simulink library "TOS_LIB"  (R2019b)
settings: Solver=VariableStepAuto  StartTime=0.0  StopTime=10.0  RelTol=1e-3
undefined symbols (not defined in the file): AEBSFunctionLib, Data, Prob_Filt
libraries: simulink x27
settings Model: Creator=GW00157303  LastModifiedBy=GW00115634
settings DataIOCC: ReturnWorkspaceOutputs=off
settings DebuggingCC: ArithmeticOperatorsInVariantConditions=warning
settings SFSimCC: SimUseLocalCustomCode=off  CustomCodeUndefinedFunction=UseInterfaceOnly
settings RTWCC: RTWUseLocalCustomCode=off
settings CodeAppCC: StateflowObjectComments=on

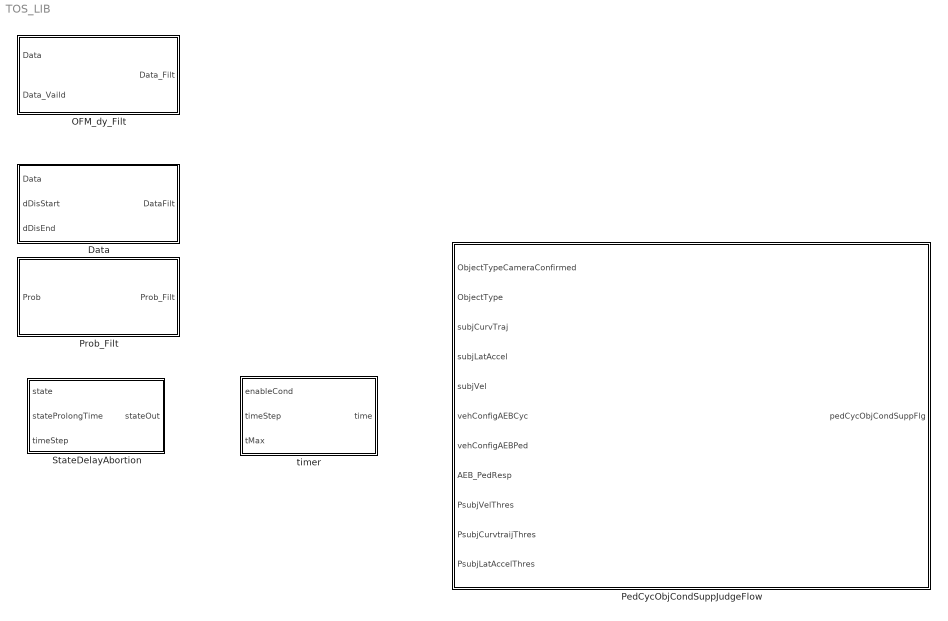
== system TOS_LIB ==
  Data : Subsystem  AncestorBlock=AEBSFunctionLib/Data
  OFM_dy_Filt : Subsystem  AncestorBlock=TOS_LIB/Prob_Filt
  PedCycObjCondSuppJudgeFlow : Subsystem  TreatAsAtomicUnit=on
  Prob_Filt : Subsystem  AncestorBlock=AEBSFunctionLib/Prob_Filt
  StateDelayAbortion : Subsystem  TreatAsAtomicUnit=on
  timer : Subsystem  TreatAsAtomicUnit=on

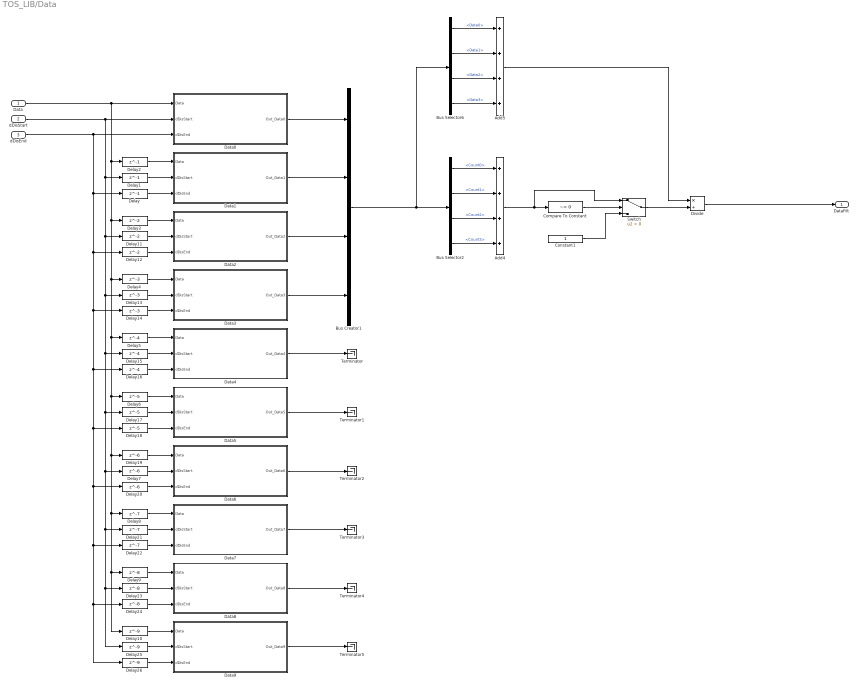
== system TOS_LIB/Data ==
  Data : Inport
  dDisStart : Inport  Port=2
  dDisEnd : Inport  Port=3
  Add4 : Sum  Inputs=++++
  Add5 : Sum  Inputs=++++
  Bus Creator1 : BusCreator  Inputs=4
  Bus Selector2 : BusSelector  OutputSignals=Out_Data0.Count0,Out_Data1.Count1,Out_Data2.Count2,Out_Data3.Count3
  Bus Selector6 : BusSelector  OutputSignals=Out_Data0.Data0,Out_Data1.Data1,Out_Data2.Data2,Out_Data3.Data3
  Compare To Constant : simulink/Logic and Bit Operations/Compare To Constant  relop=~=  const=0  OutDataTypeStr=boolean
  Constant1 : Constant  OutDataTypeStr=single
  Data0 : Subsystem
  Data1 : Subsystem
  Data2 : Subsystem
  Data3 : Subsystem
  Data4 : Subsystem
  Data5 : Subsystem
  Data6 : Subsystem
  Data7 : Subsystem
  Data8 : Subsystem
  Data9 : Subsystem
  Delay : Delay  DelayLength=1  InitialCondition=0
  Delay1 : Delay  DelayLength=1  InitialCondition=0
  Delay10 : Delay  DelayLength=9  InitialCondition=0
  Delay11 : Delay  InitialCondition=0
  Delay12 : Delay  InitialCondition=0
  Delay13 : Delay  DelayLength=3  InitialCondition=0
  Delay14 : Delay  DelayLength=3  InitialCondition=0
  Delay15 : Delay  DelayLength=4  InitialCondition=0
  Delay16 : Delay  DelayLength=4  InitialCondition=0
  Delay17 : Delay  DelayLength=5  InitialCondition=0
  Delay18 : Delay  DelayLength=5  InitialCondition=0
  Delay19 : Delay  DelayLength=6  InitialCondition=0
  Delay2 : Delay  DelayLength=1  InitialCondition=0
  Delay20 : Delay  DelayLength=6  InitialCondition=0
  Delay21 : Delay  DelayLength=7  InitialCondition=0
  Delay22 : Delay  DelayLength=7  InitialCondition=0
  Delay23 : Delay  DelayLength=8  InitialCondition=0
  Delay24 : Delay  DelayLength=8  InitialCondition=0
  Delay25 : Delay  DelayLength=9  InitialCondition=0
  Delay26 : Delay  DelayLength=9  InitialCondition=0
  Delay3 : Delay  InitialCondition=0
  Delay4 : Delay  DelayLength=3  InitialCondition=0
  Delay5 : Delay  DelayLength=4  InitialCondition=0
  Delay6 : Delay  DelayLength=5  InitialCondition=0
  Delay7 : Delay  DelayLength=6  InitialCondition=0
  Delay8 : Delay  DelayLength=7  InitialCondition=0
  Delay9 : Delay  DelayLength=8  InitialCondition=0
  Divide : Product  Inputs=*/
  Switch : Switch  Criteria=u2 > Threshold
  Terminator{,1..5} (6 alike) : Terminator
  DataFilt : Outport
  wires:
  Delay21/1 -> Data7/2(dDisStart)
  Delay18/1 -> Data5/3(dDisEnd)
  Delay9/1 -> Data8/1(Data)
  Delay22/1 -> Data7/3(dDisEnd)
  Delay23/1 -> Data8/2(dDisStart)
  Delay26/1 -> Data9/3(dDisEnd)
  Delay4/1 -> Data3/1(Data)
  Add5/1 -> Divide/1
  Delay12/1 -> Data2/3(dDisEnd)
  Delay8/1 -> Data7/1(Data)
  Data9/1(Out_Data9) -> Terminator5/1
  Data1/1(Out_Data1) -> Bus Creator1/2
  Delay7/1 -> Data6/2(dDisStart)
  dDisEnd/1 -> Data0/3(dDisEnd), Delay16/1, Delay20/1, Delay22/1, Delay26/1, Delay24/1, Delay18/1, Delay14/1, Delay12/1, Delay/1
  Delay19/1 -> Data6/1(Data)
  Delay13/1 -> Data3/2(dDisStart)
  Switch/1 -> Divide/2
  Delay14/1 -> Data3/3(dDisEnd)
  Data7/1(Out_Data7) -> Terminator3/1
  Add4/1 -> Compare To Constant/1, Switch/1
  Delay25/1 -> Data9/2(dDisStart)
  Divide/1 -> DataFilt/1
  Delay10/1 -> Data9/1(Data)
  Delay6/1 -> Data5/1(Data)
  Data4/1(Out_Data4) -> Terminator/1
  Compare To Constant/1 -> Switch/2
  Delay17/1 -> Data5/2(dDisStart)
  Delay2/1 -> Data1/1(Data)
  Delay5/1 -> Data4/1(Data)
  Delay3/1 -> Data2/1(Data)
  Delay/1 -> Data1/3(dDisEnd)
  Data3/1(Out_Data3) -> Bus Creator1/4
  Delay20/1 -> Data6/3(dDisEnd)
  Data8/1(Out_Data8) -> Terminator4/1
  Delay24/1 -> Data8/3(dDisEnd)
  dDisStart/1 -> Data0/2(dDisStart), Delay1/1, Delay25/1, Delay23/1, Delay21/1, Delay7/1, Delay17/1, Delay15/1, Delay13/1, Delay11/1
  Bus Creator1/1 -> Bus Selector2/1, Bus Selector6/1
  Data6/1(Out_Data6) -> Terminator2/1
  Delay1/1 -> Data1/2(dDisStart)
  Data5/1(Out_Data5) -> Terminator1/1
  Delay16/1 -> Data4/3(dDisEnd)
  Data2/1(Out_Data2) -> Bus Creator1/3
  Constant1/1 -> Switch/3
  Delay15/1 -> Data4/2(dDisStart)
  Data0/1(Out_Data0) -> Bus Creator1/1
  Delay11/1 -> Data2/2(dDisStart)
  Data/1 -> Delay2/1, Delay3/1, Delay6/1, Delay19/1, Delay8/1, Delay9/1, Delay10/1, Delay5/1, Delay4/1, Data0/1(Data)
  Bus Selector6/1 -> Add5/1  "<Data0>"
  Bus Selector6/2 -> Add5/2  "<Data1>"
  Bus Selector6/3 -> Add5/3  "<Data2>"
  Bus Selector6/4 -> Add5/4  "<Data3>"
  Bus Selector2/1 -> Add4/1  "<Count0>"
  Bus Selector2/2 -> Add4/2  "<Count1>"
  Bus Selector2/3 -> Add4/3  "<Count2>"
  Bus Selector2/4 -> Add4/4  "<Count3>"

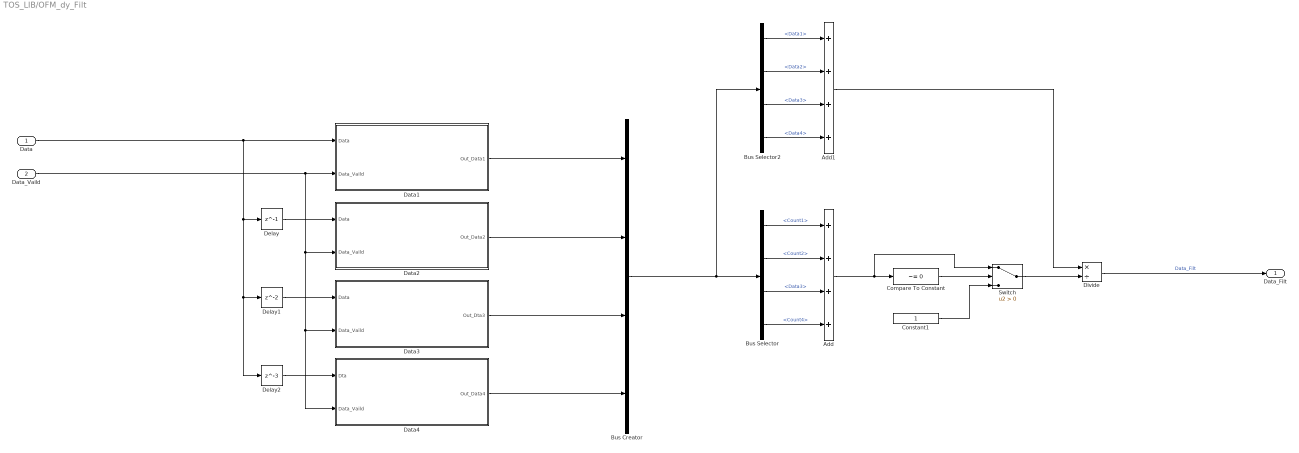
== system TOS_LIB/OFM_dy_Filt ==
  Data : Inport
  Data_Vaild : Inport  Port=2
  Add : Sum  Inputs=++++
  Add1 : Sum  Inputs=++++
  Bus Creator : BusCreator  Inputs=4
  Bus Selector : BusSelector  OutputSignals=Out_Data1.Count1,Out_Data2.Count2,Out_Data3.Data3,Out_Data4.Count4
  Bus Selector2 : BusSelector  OutputSignals=Out_Data1.Data1,Out_Data2.Data2,Out_Data3.Data3,Out_Data4.Data4
  Compare To Constant : simulink/Logic and Bit Operations/Compare To Constant  relop=~=  const=0  OutDataTypeStr=boolean
  Constant1 : Constant  OutDataTypeStr=single
  Data1 : Subsystem
  Data2 : Subsystem
  Data3 : Subsystem
  Data4 : Subsystem
  Delay : Delay  DelayLength=1  InitialCondition=0
  Delay1 : Delay  InitialCondition=0
  Delay2 : Delay  DelayLength=3  InitialCondition=0
  Divide : Product  Inputs=*/
  Switch : Switch  Criteria=u2 > Threshold
  Data_Filt : Outport
  wires:
  Bus Selector/4 -> Add/4  "<Count4>"
  Bus Selector/3 -> Add/3  "<Data3>"
  Bus Selector/2 -> Add/2  "<Count2>"
  Bus Selector/1 -> Add/1  "<Count1>"
  Bus Selector2/4 -> Add1/4  "<Data4>"
  Bus Selector2/3 -> Add1/3  "<Data3>"
  Bus Selector2/2 -> Add1/2  "<Data2>"
  Bus Selector2/1 -> Add1/1  "<Data1>"
  Divide/1 -> Data_Filt/1  "Data_Filt"
  Data3/1(Out_Dta3) -> Bus Creator/3
  Add1/1 -> Divide/1
  Data/1 -> Delay2/1, Delay1/1, Delay/1, Data1/1(Data)
  Delay2/1 -> Data4/1(Dta)
  Delay/1 -> Data2/1(Data)
  Data1/1(Out_Data1) -> Bus Creator/1
  Data2/1(Out_Data2) -> Bus Creator/2
  Bus Creator/1 -> Bus Selector2/1, Bus Selector/1
  Compare To Constant/1 -> Switch/2
  Constant1/1 -> Switch/3
  Add/1 -> Switch/1, Compare To Constant/1
  Delay1/1 -> Data3/1(Data)
  Data4/1(Out_Data4) -> Bus Creator/4
  Switch/1 -> Divide/2
  Data_Vaild/1 -> Data3/2(Data_Vaild), Data4/2(Data_Vaild), Data2/2(Data_Vaild), Data1/2(Data_Vaild)

== system TOS_LIB/PedCycObjCondSuppJudgeFlow ==
  ObjectTypeCameraConfirmed : Inport
  ObjectType : Inport  Port=2
  subjCurvTraj : Inport  Port=3
  subjLatAccel : Inport  Port=4
  subjVel : Inport  Port=5
  vehConfigAEBCyc : Inport  Port=6
  vehConfigAEBPed : Inport  Port=7
  AEB_PedResp : Inport  Port=8
  PsubjVelThres : Inport  Port=9
  PsubjCurvtraijThres : Inport  Port=10
  PsubjLatAccelThres : Inport  Port=11
  PedCycObjCondSuppJudgeFlow : Stateflow chart  TreatAsAtomicUnit=on
  pedCycObjCondSuppFlg : Outport
  wires:
  PsubjLatAccelThres/1 -> PedCycObjCondSuppJudgeFlow/11(PsubjLatAccelThres)
  PsubjCurvtraijThres/1 -> PedCycObjCondSuppJudgeFlow/10(PsubjCurvtraijThres)
  PedCycObjCondSuppJudgeFlow/1(pedCycObjCondSuppFlg) -> pedCycObjCondSuppFlg/1
  vehConfigAEBCyc/1 -> PedCycObjCondSuppJudgeFlow/6(vehConfigAEBCyc)
  subjLatAccel/1 -> PedCycObjCondSuppJudgeFlow/4(subjLatAccel)
  subjVel/1 -> PedCycObjCondSuppJudgeFlow/5(subjVel)
  ObjectType/1 -> PedCycObjCondSuppJudgeFlow/2(objType)
  AEB_PedResp/1 -> PedCycObjCondSuppJudgeFlow/8(AEB_PedResp)
  subjCurvTraj/1 -> PedCycObjCondSuppJudgeFlow/3(subjCurvTraj)
  vehConfigAEBPed/1 -> PedCycObjCondSuppJudgeFlow/7(vehConfigAEBPed)
  PsubjVelThres/1 -> PedCycObjCondSuppJudgeFlow/9(PsubjVelThres)
  ObjectTypeCameraConfirmed/1 -> PedCycObjCondSuppJudgeFlow/1(ObjectTypeCameraConfirmed)

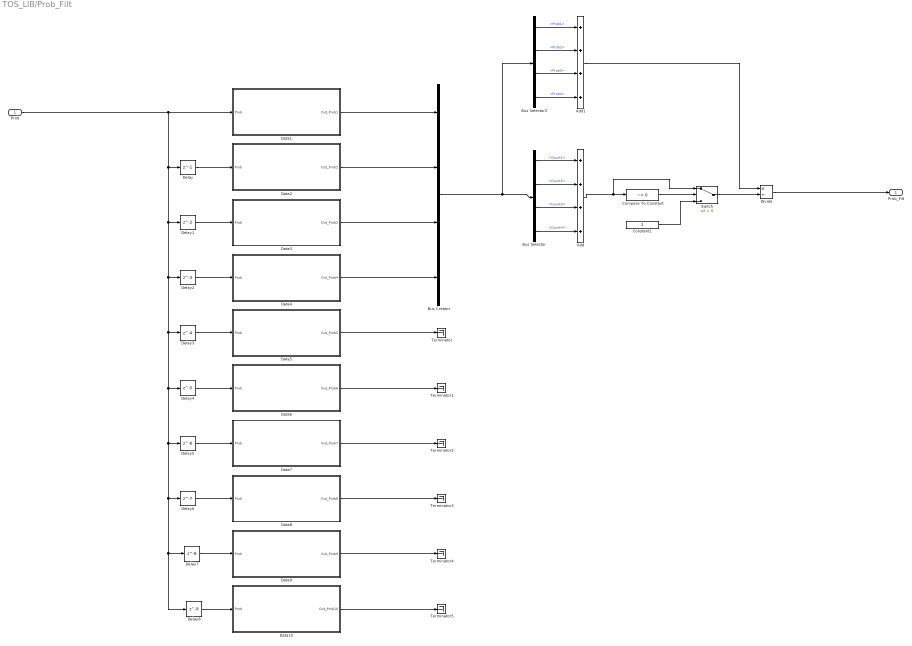
== system TOS_LIB/Prob_Filt ==
  Prob : Inport
  Add : Sum  Inputs=++++
  Add1 : Sum  Inputs=++++
  Bus Creator : BusCreator  Inputs=4
  Bus Selector : BusSelector  OutputSignals=Out_Prob1.Count1,Out_Prob2.Count2,Out_Prob3.Count3,Out_Prob4.Count4
  Bus Selector2 : BusSelector  OutputSignals=Out_Prob1.Prob1,Out_Prob2.Prob2,Out_Prob3.Prob3,Out_Prob4.Prob4
  Compare To Constant : simulink/Logic and Bit Operations/Compare To Constant  relop=~=  const=0  OutDataTypeStr=boolean
  Constant1 : Constant  OutDataTypeStr=single
  Data1 : Subsystem
  Data10 : Subsystem
  Data2 : Subsystem
  Data3 : Subsystem
  Data4 : Subsystem
  Data5 : Subsystem
  Data6 : Subsystem
  Data7 : Subsystem
  Data8 : Subsystem
  Data9 : Subsystem
  Delay : Delay  DelayLength=1  InitialCondition=0
  Delay1 : Delay  InitialCondition=0
  Delay2 : Delay  DelayLength=3  InitialCondition=0
  Delay3 : Delay  DelayLength=4  InitialCondition=0
  Delay4 : Delay  DelayLength=5  InitialCondition=0
  Delay5 : Delay  DelayLength=6  InitialCondition=0
  Delay6 : Delay  DelayLength=7  InitialCondition=0
  Delay7 : Delay  DelayLength=8  InitialCondition=0
  Delay8 : Delay  DelayLength=9  InitialCondition=0
  Divide : Product  Inputs=*/
  Switch : Switch  Criteria=u2 > Threshold
  Terminator{,1..5} (6 alike) : Terminator
  Prob_Filt : Outport
  wires:
  Switch/1 -> Divide/2
  Delay5/1 -> Data7/1(Prob)
  Delay3/1 -> Data5/1(Prob)
  Data4/1(Out_Prob4) -> Bus Creator/4
  Delay1/1 -> Data3/1(Prob)
  Delay8/1 -> Data10/1(Prob)
  Data8/1(Out_Prob8) -> Terminator3/1
  Add/1 -> Compare To Constant/1, Switch/1
  Constant1/1 -> Switch/3
  Delay6/1 -> Data8/1(Prob)
  Data10/1(Out_Prob10) -> Terminator5/1
  Compare To Constant/1 -> Switch/2
  Data5/1(Out_Prob5) -> Terminator/1
  Bus Creator/1 -> Bus Selector/1, Bus Selector2/1
  Data2/1(Out_Prob2) -> Bus Creator/2
  Data1/1(Out_Prob1) -> Bus Creator/1
  Data9/1(Out_Prob9) -> Terminator4/1
  Delay7/1 -> Data9/1(Prob)
  Delay4/1 -> Data6/1(Prob)
  Delay/1 -> Data2/1(Prob)
  Data6/1(Out_Prob6) -> Terminator1/1
  Data7/1(Out_Prob7) -> Terminator2/1
  Delay2/1 -> Data4/1(Prob)
  Prob/1 -> Delay1/1, Delay8/1, Delay7/1, Delay6/1, Delay5/1, Delay4/1, Delay3/1, Delay2/1, Delay/1, Data1/1(Prob)
  Add1/1 -> Divide/1
  Data3/1(Out_Prob3) -> Bus Creator/3
  Divide/1 -> Prob_Filt/1
  Bus Selector2/1 -> Add1/1  "<Prob1>"
  Bus Selector2/2 -> Add1/2  "<Prob2>"
  Bus Selector2/3 -> Add1/3  "<Prob3>"
  Bus Selector2/4 -> Add1/4  "<Prob4>"
  Bus Selector/1 -> Add/1  "<Count1>"
  Bus Selector/2 -> Add/2  "<Count2>"
  Bus Selector/3 -> Add/3  "<Count3>"
  Bus Selector/4 -> Add/4  "<Count4>"

== system TOS_LIB/StateDelayAbortion ==
  state : Inport
  stateProlongTime : Inport  Port=2
  timeStep : Inport  Port=3
  StateDelayAbortion : Stateflow chart  TreatAsAtomicUnit=on
  Terminator : Terminator
  Terminator1 : Terminator
  Unit Delay : UnitDelay  SampleTime=-1  HasFrameUpgradeWarning=on
  stateOut : Outport
  wires:
  StateDelayAbortion/2(stateOut) -> stateOut/1
  StateDelayAbortion/1(timeSinceLastState) -> Terminator/1  "timeSinceLastState"
  timeStep/1 -> StateDelayAbortion/4(Ts)
  stateProlongTime/1 -> StateDelayAbortion/3(stateProlongationTime)
  Unit Delay/1 -> StateDelayAbortion/2(stateK1)
  state/1 -> StateDelayAbortion/1(state), Unit Delay/1
  StateDelayAbortion/3(Flag) -> Terminator1/1  "Flag"

== system TOS_LIB/timer ==
  enableCond : Inport
  timeStep : Inport  Port=2
  tMax : Inport  Port=3
  If Action Subsystem2 : Subsystem  TreatAsAtomicUnit=on
  If Action Subsystem3 : Subsystem  TreatAsAtomicUnit=on
  If1 : If  IfExpression=u1
  Merge1 : Merge
  time : Outport
  wires:
  If1/1 -> If Action Subsystem2/Action
  If Action Subsystem2/1(time) -> Merge1/1
  If1/2 -> If Action Subsystem3/Action
  If Action Subsystem3/1(time) -> Merge1/2
  enableCond/1 -> If1/1
  timeStep/1 -> If Action Subsystem2/1(timeStep)
  Merge1/1 -> time/1  "time"
  tMax/1 -> If Action Subsystem2/2(tMax)

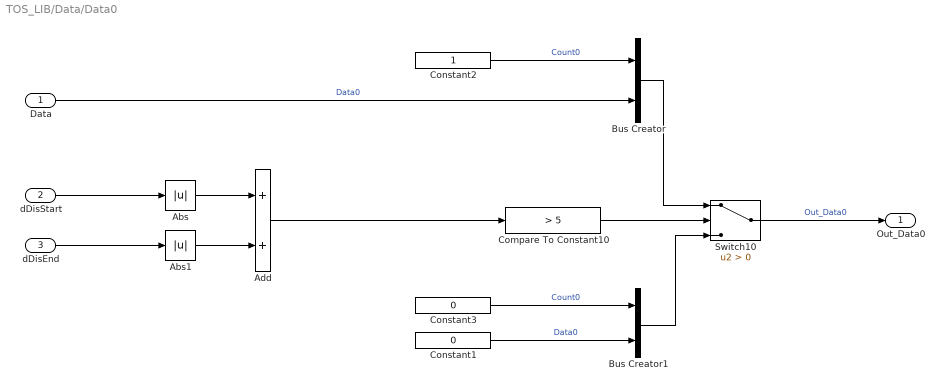
== system TOS_LIB/Data/Data0 ==
  Data : Inport
  dDisStart : Inport  Port=2
  dDisEnd : Inport  Port=3
  Abs : Abs
  Abs1 : Abs
  Add : Sum
  Bus Creator : BusCreator  Inputs=2
  Bus Creator1 : BusCreator  Inputs=2
  Compare To Constant10 : simulink/Logic and Bit Operations/Compare To Constant  relop=>  const=5  OutDataTypeStr=boolean
  Constant1 : Constant  Value=0  OutDataTypeStr=single
  Constant2 : Constant  OutDataTypeStr=uint8
  Constant3 : Constant  Value=0  OutDataTypeStr=uint8
  Switch10 : Switch  Criteria=u2 > Threshold
  Out_Data0 : Outport
  wires:
  Compare To Constant10/1 -> Switch10/2
  Constant3/1 -> Bus Creator1/1  "Count0"
  Constant1/1 -> Bus Creator1/2  "Data0"
  Switch10/1 -> Out_Data0/1  "Out_Data0"
  Constant2/1 -> Bus Creator/1  "Count0"
  Bus Creator1/1 -> Switch10/3
  Bus Creator/1 -> Switch10/1
  Add/1 -> Compare To Constant10/1
  dDisStart/1 -> Abs/1
  dDisEnd/1 -> Abs1/1
  Abs/1 -> Add/1
  Abs1/1 -> Add/2
  Data/1 -> Bus Creator/2  "Data0"

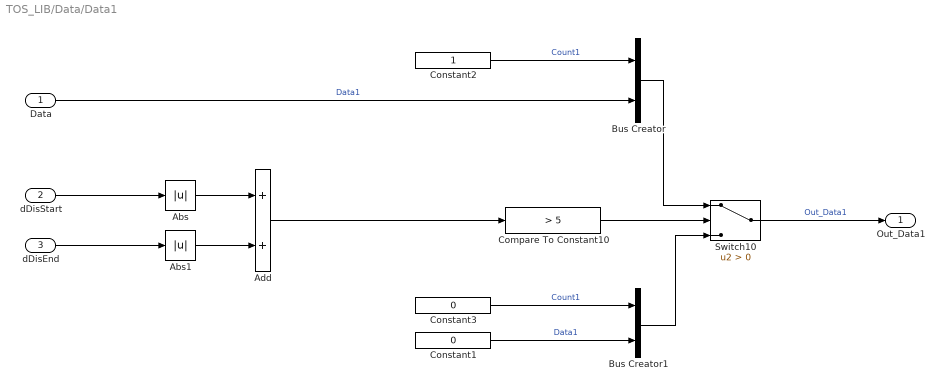
== system TOS_LIB/Data/Data1 ==
  Data : Inport
  dDisStart : Inport  Port=2
  dDisEnd : Inport  Port=3
  Abs : Abs
  Abs1 : Abs
  Add : Sum
  Bus Creator : BusCreator  Inputs=2
  Bus Creator1 : BusCreator  Inputs=2
  Compare To Constant10 : simulink/Logic and Bit Operations/Compare To Constant  relop=>  const=5  OutDataTypeStr=boolean
  Constant1 : Constant  Value=0  OutDataTypeStr=single
  Constant2 : Constant  OutDataTypeStr=uint8
  Constant3 : Constant  Value=0  OutDataTypeStr=uint8
  Switch10 : Switch  Criteria=u2 > Threshold
  Out_Data1 : Outport
  wires:
  Data/1 -> Bus Creator/2  "Data1"
  Abs1/1 -> Add/2
  Abs/1 -> Add/1
  dDisEnd/1 -> Abs1/1
  dDisStart/1 -> Abs/1
  Add/1 -> Compare To Constant10/1
  Bus Creator/1 -> Switch10/1
  Bus Creator1/1 -> Switch10/3
  Constant2/1 -> Bus Creator/1  "Count1"
  Switch10/1 -> Out_Data1/1  "Out_Data1"
  Constant1/1 -> Bus Creator1/2  "Data1"
  Constant3/1 -> Bus Creator1/1  "Count1"
  Compare To Constant10/1 -> Switch10/2

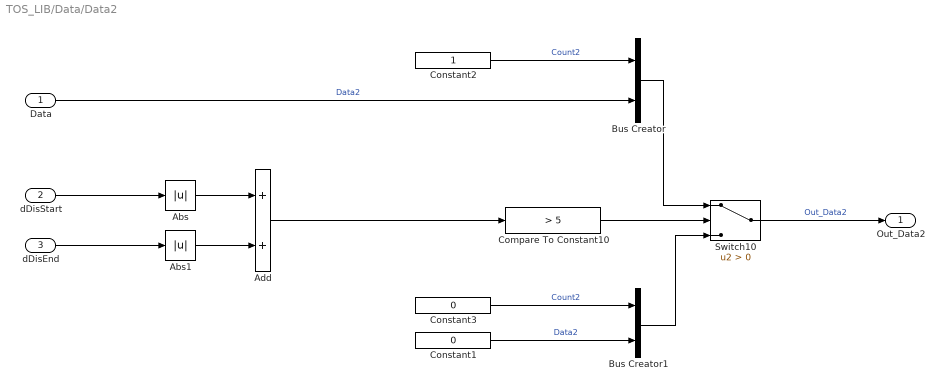
== system TOS_LIB/Data/Data2 ==
  Data : Inport
  dDisStart : Inport  Port=2
  dDisEnd : Inport  Port=3
  Abs : Abs
  Abs1 : Abs
  Add : Sum
  Bus Creator : BusCreator  Inputs=2
  Bus Creator1 : BusCreator  Inputs=2
  Compare To Constant10 : simulink/Logic and Bit Operations/Compare To Constant  relop=>  const=5  OutDataTypeStr=boolean
  Constant1 : Constant  Value=0  OutDataTypeStr=single
  Constant2 : Constant  OutDataTypeStr=uint8
  Constant3 : Constant  Value=0  OutDataTypeStr=uint8
  Switch10 : Switch  Criteria=u2 > Threshold
  Out_Data2 : Outport
  wires:
  Compare To Constant10/1 -> Switch10/2
  Constant3/1 -> Bus Creator1/1  "Count2"
  Constant1/1 -> Bus Creator1/2  "Data2"
  Switch10/1 -> Out_Data2/1  "Out_Data2"
  Constant2/1 -> Bus Creator/1  "Count2"
  Bus Creator1/1 -> Switch10/3
  Bus Creator/1 -> Switch10/1
  Add/1 -> Compare To Constant10/1
  dDisStart/1 -> Abs/1
  dDisEnd/1 -> Abs1/1
  Abs/1 -> Add/1
  Abs1/1 -> Add/2
  Data/1 -> Bus Creator/2  "Data2"

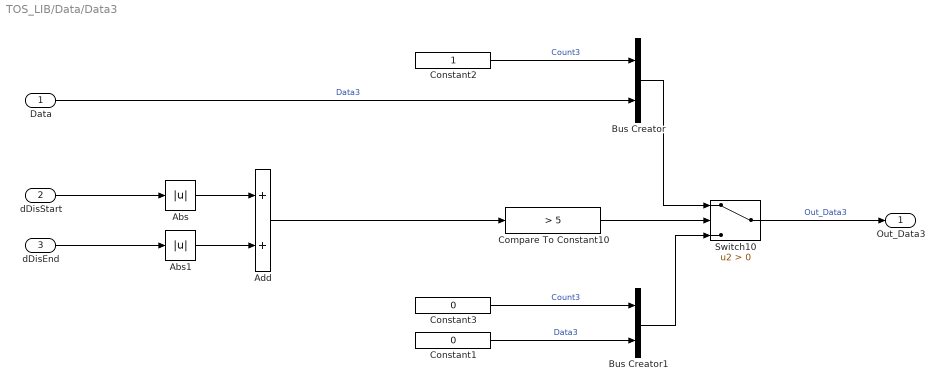
== system TOS_LIB/Data/Data3 ==
  Data : Inport
  dDisStart : Inport  Port=2
  dDisEnd : Inport  Port=3
  Abs : Abs
  Abs1 : Abs
  Add : Sum
  Bus Creator : BusCreator  Inputs=2
  Bus Creator1 : BusCreator  Inputs=2
  Compare To Constant10 : simulink/Logic and Bit Operations/Compare To Constant  relop=>  const=5  OutDataTypeStr=boolean
  Constant1 : Constant  Value=0  OutDataTypeStr=single
  Constant2 : Constant  OutDataTypeStr=uint8
  Constant3 : Constant  Value=0  OutDataTypeStr=uint8
  Switch10 : Switch  Criteria=u2 > Threshold
  Out_Data3 : Outport
  wires:
  Compare To Constant10/1 -> Switch10/2
  Constant3/1 -> Bus Creator1/1  "Count3"
  Constant1/1 -> Bus Creator1/2  "Data3"
  Switch10/1 -> Out_Data3/1  "Out_Data3"
  Constant2/1 -> Bus Creator/1  "Count3"
  Bus Creator1/1 -> Switch10/3
  Bus Creator/1 -> Switch10/1
  Add/1 -> Compare To Constant10/1
  dDisStart/1 -> Abs/1
  dDisEnd/1 -> Abs1/1
  Abs/1 -> Add/1
  Abs1/1 -> Add/2
  Data/1 -> Bus Creator/2  "Data3"

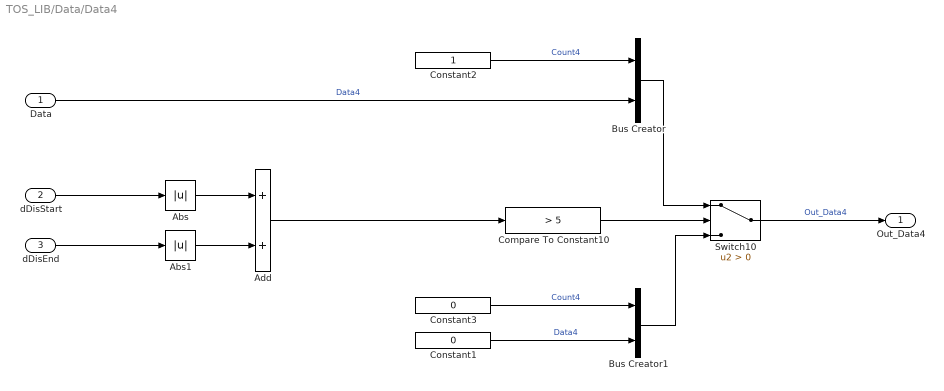
== system TOS_LIB/Data/Data4 ==
  Data : Inport
  dDisStart : Inport  Port=2
  dDisEnd : Inport  Port=3
  Abs : Abs
  Abs1 : Abs
  Add : Sum
  Bus Creator : BusCreator  Inputs=2
  Bus Creator1 : BusCreator  Inputs=2
  Compare To Constant10 : simulink/Logic and Bit Operations/Compare To Constant  relop=>  const=5  OutDataTypeStr=boolean
  Constant1 : Constant  Value=0  OutDataTypeStr=single
  Constant2 : Constant  OutDataTypeStr=uint8
  Constant3 : Constant  Value=0  OutDataTypeStr=uint8
  Switch10 : Switch  Criteria=u2 > Threshold
  Out_Data4 : Outport
  wires:
  Data/1 -> Bus Creator/2  "Data4"
  Abs1/1 -> Add/2
  Abs/1 -> Add/1
  dDisEnd/1 -> Abs1/1
  dDisStart/1 -> Abs/1
  Add/1 -> Compare To Constant10/1
  Bus Creator/1 -> Switch10/1
  Bus Creator1/1 -> Switch10/3
  Constant2/1 -> Bus Creator/1  "Count4"
  Switch10/1 -> Out_Data4/1  "Out_Data4"
  Constant1/1 -> Bus Creator1/2  "Data4"
  Constant3/1 -> Bus Creator1/1  "Count4"
  Compare To Constant10/1 -> Switch10/2

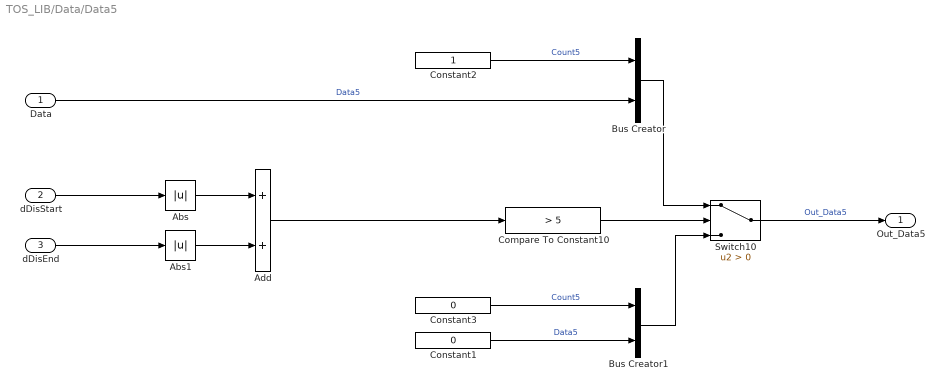
== system TOS_LIB/Data/Data5 ==
  Data : Inport
  dDisStart : Inport  Port=2
  dDisEnd : Inport  Port=3
  Abs : Abs
  Abs1 : Abs
  Add : Sum
  Bus Creator : BusCreator  Inputs=2
  Bus Creator1 : BusCreator  Inputs=2
  Compare To Constant10 : simulink/Logic and Bit Operations/Compare To Constant  relop=>  const=5  OutDataTypeStr=boolean
  Constant1 : Constant  Value=0  OutDataTypeStr=single
  Constant2 : Constant  OutDataTypeStr=uint8
  Constant3 : Constant  Value=0  OutDataTypeStr=uint8
  Switch10 : Switch  Criteria=u2 > Threshold
  Out_Data5 : Outport
  wires:
  Compare To Constant10/1 -> Switch10/2
  Constant3/1 -> Bus Creator1/1  "Count5"
  Constant1/1 -> Bus Creator1/2  "Data5"
  Switch10/1 -> Out_Data5/1  "Out_Data5"
  Constant2/1 -> Bus Creator/1  "Count5"
  Bus Creator1/1 -> Switch10/3
  Bus Creator/1 -> Switch10/1
  Add/1 -> Compare To Constant10/1
  dDisStart/1 -> Abs/1
  dDisEnd/1 -> Abs1/1
  Abs/1 -> Add/1
  Abs1/1 -> Add/2
  Data/1 -> Bus Creator/2  "Data5"

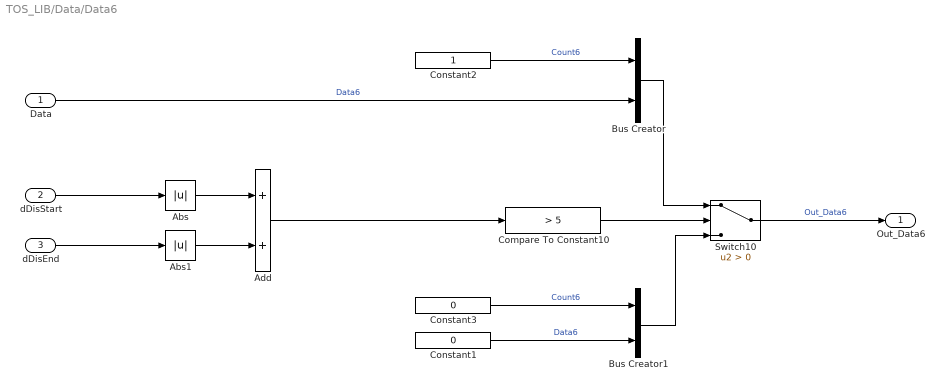
== system TOS_LIB/Data/Data6 ==
  Data : Inport
  dDisStart : Inport  Port=2
  dDisEnd : Inport  Port=3
  Abs : Abs
  Abs1 : Abs
  Add : Sum
  Bus Creator : BusCreator  Inputs=2
  Bus Creator1 : BusCreator  Inputs=2
  Compare To Constant10 : simulink/Logic and Bit Operations/Compare To Constant  relop=>  const=5  OutDataTypeStr=boolean
  Constant1 : Constant  Value=0  OutDataTypeStr=single
  Constant2 : Constant  OutDataTypeStr=uint8
  Constant3 : Constant  Value=0  OutDataTypeStr=uint8
  Switch10 : Switch  Criteria=u2 > Threshold
  Out_Data6 : Outport
  wires:
  Data/1 -> Bus Creator/2  "Data6"
  Abs1/1 -> Add/2
  Abs/1 -> Add/1
  dDisEnd/1 -> Abs1/1
  dDisStart/1 -> Abs/1
  Add/1 -> Compare To Constant10/1
  Bus Creator/1 -> Switch10/1
  Bus Creator1/1 -> Switch10/3
  Constant2/1 -> Bus Creator/1  "Count6"
  Switch10/1 -> Out_Data6/1  "Out_Data6"
  Constant1/1 -> Bus Creator1/2  "Data6"
  Constant3/1 -> Bus Creator1/1  "Count6"
  Compare To Constant10/1 -> Switch10/2

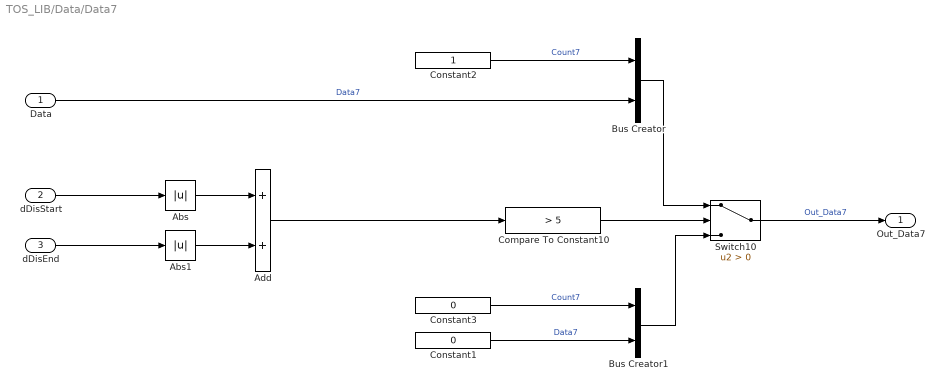
== system TOS_LIB/Data/Data7 ==
  Data : Inport
  dDisStart : Inport  Port=2
  dDisEnd : Inport  Port=3
  Abs : Abs
  Abs1 : Abs
  Add : Sum
  Bus Creator : BusCreator  Inputs=2
  Bus Creator1 : BusCreator  Inputs=2
  Compare To Constant10 : simulink/Logic and Bit Operations/Compare To Constant  relop=>  const=5  OutDataTypeStr=boolean
  Constant1 : Constant  Value=0  OutDataTypeStr=single
  Constant2 : Constant  OutDataTypeStr=uint8
  Constant3 : Constant  Value=0  OutDataTypeStr=uint8
  Switch10 : Switch  Criteria=u2 > Threshold
  Out_Data7 : Outport
  wires:
  Data/1 -> Bus Creator/2  "Data7"
  Abs1/1 -> Add/2
  Abs/1 -> Add/1
  dDisEnd/1 -> Abs1/1
  dDisStart/1 -> Abs/1
  Add/1 -> Compare To Constant10/1
  Bus Creator/1 -> Switch10/1
  Bus Creator1/1 -> Switch10/3
  Constant2/1 -> Bus Creator/1  "Count7"
  Switch10/1 -> Out_Data7/1  "Out_Data7"
  Constant1/1 -> Bus Creator1/2  "Data7"
  Constant3/1 -> Bus Creator1/1  "Count7"
  Compare To Constant10/1 -> Switch10/2

== system TOS_LIB/Data/Data8 ==
  Data : Inport
  dDisStart : Inport  Port=2
  dDisEnd : Inport  Port=3
  Abs : Abs
  Abs1 : Abs
  Add : Sum
  Bus Creator : BusCreator  Inputs=2
  Bus Creator1 : BusCreator  Inputs=2
  Compare To Constant10 : simulink/Logic and Bit Operations/Compare To Constant  relop=>  const=5  OutDataTypeStr=boolean
  Constant1 : Constant  Value=0  OutDataTypeStr=single
  Constant2 : Constant  OutDataTypeStr=uint8
  Constant3 : Constant  Value=0  OutDataTypeStr=uint8
  Switch10 : Switch  Criteria=u2 > Threshold
  Out_Data8 : Outport
  wires:
  Compare To Constant10/1 -> Switch10/2
  Constant3/1 -> Bus Creator1/1  "Count8"
  Constant1/1 -> Bus Creator1/2  "Data8"
  Switch10/1 -> Out_Data8/1  "Out_Data8"
  Constant2/1 -> Bus Creator/1  "Count8"
  Bus Creator1/1 -> Switch10/3
  Bus Creator/1 -> Switch10/1
  Add/1 -> Compare To Constant10/1
  dDisStart/1 -> Abs/1
  dDisEnd/1 -> Abs1/1
  Abs/1 -> Add/1
  Abs1/1 -> Add/2
  Data/1 -> Bus Creator/2  "Data8"

== system TOS_LIB/Data/Data9 ==
  Data : Inport
  dDisStart : Inport  Port=2
  dDisEnd : Inport  Port=3
  Abs : Abs
  Abs1 : Abs
  Add : Sum
  Bus Creator : BusCreator  Inputs=2
  Bus Creator1 : BusCreator  Inputs=2
  Compare To Constant10 : simulink/Logic and Bit Operations/Compare To Constant  relop=>  const=5  OutDataTypeStr=boolean
  Constant1 : Constant  Value=0  OutDataTypeStr=single
  Constant2 : Constant  OutDataTypeStr=uint8
  Constant3 : Constant  Value=0  OutDataTypeStr=uint8
  Switch10 : Switch  Criteria=u2 > Threshold
  Out_Data9 : Outport
  wires:
  Compare To Constant10/1 -> Switch10/2
  Constant3/1 -> Bus Creator1/1  "Count9"
  Constant1/1 -> Bus Creator1/2  "Data9"
  Switch10/1 -> Out_Data9/1  "Out_Data9"
  Constant2/1 -> Bus Creator/1  "Count9"
  Bus Creator1/1 -> Switch10/3
  Bus Creator/1 -> Switch10/1
  Add/1 -> Compare To Constant10/1
  dDisStart/1 -> Abs/1
  dDisEnd/1 -> Abs1/1
  Abs/1 -> Add/1
  Abs1/1 -> Add/2
  Data/1 -> Bus Creator/2  "Data9"

== system TOS_LIB/OFM_dy_Filt/Data1 ==
  Data : Inport
  Data_Vaild : Inport  Port=2
  Bus Creator : BusCreator  Inputs=2
  Bus Creator1 : BusCreator  Inputs=2
  Compare To Constant10 : simulink/Logic and Bit Operations/Compare To Constant  relop=~=  const=0  OutDataTypeStr=boolean
  Constant1 : Constant  Value=0  OutDataTypeStr=single
  Constant2 : Constant  OutDataTypeStr=uint8
  Constant3 : Constant  Value=0  OutDataTypeStr=uint8
  Switch10 : Switch  Criteria=u2 > Threshold
  Out_Data1 : Outport
  wires:
  Compare To Constant10/1 -> Switch10/2
  Constant3/1 -> Bus Creator1/1  "Count1"
  Constant1/1 -> Bus Creator1/2  "Data1"
  Switch10/1 -> Out_Data1/1  "Out_Data1"
  Constant2/1 -> Bus Creator/1  "Count1"
  Bus Creator1/1 -> Switch10/3
  Bus Creator/1 -> Switch10/1
  Data/1 -> Bus Creator/2  "Data1"
  Data_Vaild/1 -> Compare To Constant10/1

== system TOS_LIB/OFM_dy_Filt/Data2 ==
  Data : Inport
  Data_Vaild : Inport  Port=2
  Bus Creator : BusCreator  Inputs=2
  Bus Creator1 : BusCreator  Inputs=2
  Compare To Constant10 : simulink/Logic and Bit Operations/Compare To Constant  relop=~=  const=0  OutDataTypeStr=boolean
  Constant1 : Constant  Value=0  OutDataTypeStr=single
  Constant2 : Constant  OutDataTypeStr=uint8
  Constant3 : Constant  Value=0  OutDataTypeStr=uint8
  Switch10 : Switch  Criteria=u2 > Threshold
  Out_Data2 : Outport
  wires:
  Data_Vaild/1 -> Compare To Constant10/1
  Bus Creator/1 -> Switch10/1
  Bus Creator1/1 -> Switch10/3
  Constant2/1 -> Bus Creator/1  "Count2"
  Switch10/1 -> Out_Data2/1  "Out_Data2"
  Constant1/1 -> Bus Creator1/2  "Data2"
  Constant3/1 -> Bus Creator1/1  "Count2"
  Compare To Constant10/1 -> Switch10/2
  Data/1 -> Bus Creator/2  "Data2"

== system TOS_LIB/OFM_dy_Filt/Data3 ==
  Data : Inport
  Data_Vaild : Inport  Port=2
  Bus Creator : BusCreator  Inputs=2
  Bus Creator1 : BusCreator  Inputs=2
  Compare To Constant10 : simulink/Logic and Bit Operations/Compare To Constant  relop=~=  const=0  OutDataTypeStr=boolean
  Constant1 : Constant  Value=0  OutDataTypeStr=single
  Constant2 : Constant  OutDataTypeStr=uint8
  Constant3 : Constant  Value=0  OutDataTypeStr=uint8
  Switch10 : Switch  Criteria=u2 > Threshold
  Out_Dta3 : Outport
  wires:
  Bus Creator/1 -> Switch10/1
  Bus Creator1/1 -> Switch10/3
  Constant2/1 -> Bus Creator/1  "Count3"
  Switch10/1 -> Out_Dta3/1  "Out_Data3"
  Constant1/1 -> Bus Creator1/2  "Data3"
  Constant3/1 -> Bus Creator1/1  "Count3"
  Compare To Constant10/1 -> Switch10/2
  Data/1 -> Bus Creator/2  "Data3"
  Data_Vaild/1 -> Compare To Constant10/1  "Dta2"

== system TOS_LIB/OFM_dy_Filt/Data4 ==
  Dta : Inport
  Data_Vaild : Inport  Port=2
  Bus Creator : BusCreator  Inputs=2
  Bus Creator1 : BusCreator  Inputs=2
  Compare To Constant10 : simulink/Logic and Bit Operations/Compare To Constant  relop=~=  const=0  OutDataTypeStr=boolean
  Constant1 : Constant  Value=0  OutDataTypeStr=single
  Constant2 : Constant  OutDataTypeStr=uint8
  Constant3 : Constant  Value=0  OutDataTypeStr=uint8
  Switch10 : Switch  Criteria=u2 > Threshold
  Out_Data4 : Outport
  wires:
  Compare To Constant10/1 -> Switch10/2
  Constant3/1 -> Bus Creator1/1  "Count4"
  Constant1/1 -> Bus Creator1/2  "Data4"
  Switch10/1 -> Out_Data4/1  "Out_Data4"
  Constant2/1 -> Bus Creator/1  "Count4"
  Bus Creator1/1 -> Switch10/3
  Bus Creator/1 -> Switch10/1
  Dta/1 -> Bus Creator/2  "Data4"
  Data_Vaild/1 -> Compare To Constant10/1

== system TOS_LIB/Prob_Filt/Data1 ==
  Prob : Inport
  Bus Creator : BusCreator  Inputs=2
  Bus Creator1 : BusCreator  Inputs=2
  Compare To Constant10 : simulink/Logic and Bit Operations/Compare To Constant  relop=>=  const=0.001  OutDataTypeStr=boolean
  Constant1 : Constant  Value=0  OutDataTypeStr=single
  Constant2 : Constant  OutDataTypeStr=uint8
  Constant3 : Constant  Value=0  OutDataTypeStr=uint8
  Switch10 : Switch  Criteria=u2 > Threshold
  Out_Prob1 : Outport
  wires:
  Prob/1 -> Bus Creator/2, Compare To Constant10/1  "Prob1"
  Bus Creator/1 -> Switch10/1
  Bus Creator1/1 -> Switch10/3
  Constant2/1 -> Bus Creator/1  "Count1"
  Switch10/1 -> Out_Prob1/1  "Out_Prob1"
  Constant1/1 -> Bus Creator1/2  "Prob1"
  Constant3/1 -> Bus Creator1/1  "Count1"
  Compare To Constant10/1 -> Switch10/2

== system TOS_LIB/Prob_Filt/Data10 ==
  Prob : Inport
  Bus Creator : BusCreator  Inputs=2
  Bus Creator1 : BusCreator  Inputs=2
  Compare To Constant10 : simulink/Logic and Bit Operations/Compare To Constant  relop=>=  const=0.001  OutDataTypeStr=boolean
  Constant1 : Constant  Value=0  OutDataTypeStr=single
  Constant2 : Constant  OutDataTypeStr=uint8
  Constant3 : Constant  Value=0  OutDataTypeStr=uint8
  Switch10 : Switch  Criteria=u2 > Threshold
  Out_Prob10 : Outport
  wires:
  Prob/1 -> Bus Creator/2, Compare To Constant10/1  "Prob10"
  Bus Creator/1 -> Switch10/1
  Bus Creator1/1 -> Switch10/3
  Constant2/1 -> Bus Creator/1  "Count10"
  Switch10/1 -> Out_Prob10/1  "Out_Prob10"
  Constant1/1 -> Bus Creator1/2  "Prob10"
  Constant3/1 -> Bus Creator1/1  "Count10"
  Compare To Constant10/1 -> Switch10/2

== system TOS_LIB/Prob_Filt/Data2 ==
  Prob : Inport
  Bus Creator : BusCreator  Inputs=2
  Bus Creator1 : BusCreator  Inputs=2
  Compare To Constant10 : simulink/Logic and Bit Operations/Compare To Constant  relop=>=  const=0.001  OutDataTypeStr=boolean
  Constant1 : Constant  Value=0  OutDataTypeStr=single
  Constant2 : Constant  OutDataTypeStr=uint8
  Constant3 : Constant  Value=0  OutDataTypeStr=uint8
  Switch10 : Switch  Criteria=u2 > Threshold
  Out_Prob2 : Outport
  wires:
  Compare To Constant10/1 -> Switch10/2
  Constant3/1 -> Bus Creator1/1  "Count2"
  Constant1/1 -> Bus Creator1/2  "Prob2"
  Switch10/1 -> Out_Prob2/1  "Out_Prob2"
  Constant2/1 -> Bus Creator/1  "Count2"
  Bus Creator1/1 -> Switch10/3
  Bus Creator/1 -> Switch10/1
  Prob/1 -> Compare To Constant10/1, Bus Creator/2  "Prob2"

== system TOS_LIB/Prob_Filt/Data3 ==
  Prob : Inport
  Bus Creator : BusCreator  Inputs=2
  Bus Creator1 : BusCreator  Inputs=2
  Compare To Constant10 : simulink/Logic and Bit Operations/Compare To Constant  relop=>=  const=0.001  OutDataTypeStr=boolean
  Constant1 : Constant  Value=0  OutDataTypeStr=single
  Constant2 : Constant  OutDataTypeStr=uint8
  Constant3 : Constant  Value=0  OutDataTypeStr=uint8
  Switch10 : Switch  Criteria=u2 > Threshold
  Out_Prob3 : Outport
  wires:
  Compare To Constant10/1 -> Switch10/2
  Constant3/1 -> Bus Creator1/1  "Count3"
  Constant1/1 -> Bus Creator1/2  "Prob3"
  Switch10/1 -> Out_Prob3/1  "Out_Prob3"
  Constant2/1 -> Bus Creator/1  "Count3"
  Bus Creator1/1 -> Switch10/3
  Bus Creator/1 -> Switch10/1
  Prob/1 -> Compare To Constant10/1, Bus Creator/2  "Prob3"

== system TOS_LIB/Prob_Filt/Data4 ==
  Prob : Inport
  Bus Creator : BusCreator  Inputs=2
  Bus Creator1 : BusCreator  Inputs=2
  Compare To Constant10 : simulink/Logic and Bit Operations/Compare To Constant  relop=>=  const=0.001  OutDataTypeStr=boolean
  Constant1 : Constant  Value=0  OutDataTypeStr=single
  Constant2 : Constant  OutDataTypeStr=uint8
  Constant3 : Constant  Value=0  OutDataTypeStr=uint8
  Switch10 : Switch  Criteria=u2 > Threshold
  Out_Prob4 : Outport
  wires:
  Prob/1 -> Bus Creator/2, Compare To Constant10/1  "Prob4"
  Bus Creator/1 -> Switch10/1
  Bus Creator1/1 -> Switch10/3
  Constant2/1 -> Bus Creator/1  "Count4"
  Switch10/1 -> Out_Prob4/1  "Out_Prob4"
  Constant1/1 -> Bus Creator1/2  "Prob4"
  Constant3/1 -> Bus Creator1/1  "Count4"
  Compare To Constant10/1 -> Switch10/2

== system TOS_LIB/Prob_Filt/Data5 ==
  Prob : Inport
  Bus Creator : BusCreator  Inputs=2
  Bus Creator1 : BusCreator  Inputs=2
  Compare To Constant10 : simulink/Logic and Bit Operations/Compare To Constant  relop=>=  const=0.001  OutDataTypeStr=boolean
  Constant1 : Constant  Value=0  OutDataTypeStr=single
  Constant2 : Constant  OutDataTypeStr=uint8
  Constant3 : Constant  Value=0  OutDataTypeStr=uint8
  Switch10 : Switch  Criteria=u2 > Threshold
  Out_Prob5 : Outport
  wires:
  Compare To Constant10/1 -> Switch10/2
  Constant3/1 -> Bus Creator1/1  "Count5"
  Constant1/1 -> Bus Creator1/2  "Prob5"
  Switch10/1 -> Out_Prob5/1  "Out_Prob5"
  Constant2/1 -> Bus Creator/1  "Count5"
  Bus Creator1/1 -> Switch10/3
  Bus Creator/1 -> Switch10/1
  Prob/1 -> Compare To Constant10/1, Bus Creator/2  "Prob5"

== system TOS_LIB/Prob_Filt/Data6 ==
  Prob : Inport
  Bus Creator : BusCreator  Inputs=2
  Bus Creator1 : BusCreator  Inputs=2
  Compare To Constant10 : simulink/Logic and Bit Operations/Compare To Constant  relop=>=  const=0.001  OutDataTypeStr=boolean
  Constant1 : Constant  Value=0  OutDataTypeStr=single
  Constant2 : Constant  OutDataTypeStr=uint8
  Constant3 : Constant  Value=0  OutDataTypeStr=uint8
  Switch10 : Switch  Criteria=u2 > Threshold
  Out_Prob6 : Outport
  wires:
  Prob/1 -> Bus Creator/2, Compare To Constant10/1  "Prob6"
  Bus Creator/1 -> Switch10/1
  Bus Creator1/1 -> Switch10/3
  Constant2/1 -> Bus Creator/1  "Count6"
  Switch10/1 -> Out_Prob6/1  "Out_Prob6"
  Constant1/1 -> Bus Creator1/2  "Prob6"
  Constant3/1 -> Bus Creator1/1  "Count6"
  Compare To Constant10/1 -> Switch10/2

== system TOS_LIB/Prob_Filt/Data7 ==
  Prob : Inport
  Bus Creator : BusCreator  Inputs=2
  Bus Creator1 : BusCreator  Inputs=2
  Compare To Constant10 : simulink/Logic and Bit Operations/Compare To Constant  relop=>=  const=0.001  OutDataTypeStr=boolean
  Constant1 : Constant  Value=0  OutDataTypeStr=single
  Constant2 : Constant  OutDataTypeStr=uint8
  Constant3 : Constant  Value=0  OutDataTypeStr=uint8
  Switch10 : Switch  Criteria=u2 > Threshold
  Out_Prob7 : Outport
  wires:
  Prob/1 -> Bus Creator/2, Compare To Constant10/1  "Prob7"
  Bus Creator/1 -> Switch10/1
  Bus Creator1/1 -> Switch10/3
  Constant2/1 -> Bus Creator/1  "Count7"
  Switch10/1 -> Out_Prob7/1  "Out_Prob7"
  Constant1/1 -> Bus Creator1/2  "Prob7"
  Constant3/1 -> Bus Creator1/1  "Count7"
  Compare To Constant10/1 -> Switch10/2

== system TOS_LIB/Prob_Filt/Data8 ==
  Prob : Inport
  Bus Creator : BusCreator  Inputs=2
  Bus Creator1 : BusCreator  Inputs=2
  Compare To Constant10 : simulink/Logic and Bit Operations/Compare To Constant  relop=>=  const=0.001  OutDataTypeStr=boolean
  Constant1 : Constant  Value=0  OutDataTypeStr=single
  Constant2 : Constant  OutDataTypeStr=uint8
  Constant3 : Constant  Value=0  OutDataTypeStr=uint8
  Switch10 : Switch  Criteria=u2 > Threshold
  Out_Prob8 : Outport
  wires:
  Compare To Constant10/1 -> Switch10/2
  Constant3/1 -> Bus Creator1/1  "Count8"
  Constant1/1 -> Bus Creator1/2  "Prob8"
  Switch10/1 -> Out_Prob8/1  "Out_Prob8"
  Constant2/1 -> Bus Creator/1  "Count8"
  Bus Creator1/1 -> Switch10/3
  Bus Creator/1 -> Switch10/1
  Prob/1 -> Compare To Constant10/1, Bus Creator/2  "Prob8"

== system TOS_LIB/Prob_Filt/Data9 ==
  Prob : Inport
  Bus Creator : BusCreator  Inputs=2
  Bus Creator1 : BusCreator  Inputs=2
  Compare To Constant10 : simulink/Logic and Bit Operations/Compare To Constant  relop=>=  const=0.001  OutDataTypeStr=boolean
  Constant1 : Constant  Value=0  OutDataTypeStr=single
  Constant2 : Constant  OutDataTypeStr=uint8
  Constant3 : Constant  Value=0  OutDataTypeStr=uint8
  Switch10 : Switch  Criteria=u2 > Threshold
  Out_Prob9 : Outport
  wires:
  Compare To Constant10/1 -> Switch10/2
  Constant3/1 -> Bus Creator1/1  "Count9"
  Constant1/1 -> Bus Creator1/2  "Prob9"
  Switch10/1 -> Out_Prob9/1  "Out_Prob9"
  Constant2/1 -> Bus Creator/1  "Count9"
  Bus Creator1/1 -> Switch10/3
  Bus Creator/1 -> Switch10/1
  Prob/1 -> Compare To Constant10/1, Bus Creator/2  "Prob9"

== system TOS_LIB/timer/If Action Subsystem2 ==
  timeStep : Inport
  tMax : Inport  Port=2
  Action Port : ActionPort  InitializeStates=reset
  Add : Sum
  MinMax : MinMax  Inputs=2
  Unit Delay : UnitDelay  SampleTime=-1  HasFrameUpgradeWarning=on
      settings: AttributesFormatString=InitialCondition:%<InitialCondition>
  time : Outport
  wires:
  Add/1 -> Unit Delay/1, MinMax/1
  tMax/1 -> MinMax/2
  MinMax/1 -> time/1
  timeStep/1 -> Add/1
  Unit Delay/1 -> Add/2

== system TOS_LIB/timer/If Action Subsystem3 ==
  Action Port : ActionPort
  Constant : Constant  Value=0
  time : Outport
  wires:
  Constant/1 -> time/1

== stateflow chart TOS_LIB/PedCycObjCondSuppJudgeFlow/PedCycObjCondSuppJudgeFlow ==
  (default) -> (junction 2)
  (junction 2) -> (junction 3) [order 1] : [objType == ObjectType.PEDESTRIAN ||...
      | objType == ObjectType.BICYCLE]
  (junction 2) -> (junction 7) [order 2] : {
      | 	pedCycObjCondSuppFlg = false;
      | }
  (junction 3) -> (junction 5)
  (junction 5) -> (junction 9) [order 1] : [abs(subjCurvTraj) > PsubjCurvtraijThres ||...
      | abs(subjLatAccel) > PsubjLatAccelThres]
  (junction 5) -> (junction 13) [order 2] : {
      | 	subjDrvCondSuppFlg = false;
      | }
  (junction 9) -> (junction 11) : {
      | 	subjDrvCondSuppFlg = true;
      | }
  (junction 11) -> (junction 13)
  (junction 13) -> (junction 16)
  (junction 16) -> (junction 18) [order 1] : [subjVel > PsubjVelThres ||...
      | ObjectTypeCameraConfirmed == false ||...
      | subjDrvCondSuppFlg == true || ...
      | AEB_PedResp == CNSwtOFF ||...
      | vehConfigAEBPed == false ||...
      | vehConfigAEBCyc == false]
  (junction 16) -> (junction 22) [order 2] : {
      | 	pedCycObjCondSuppFlg = false;
      | }
  (junction 18) -> (junction 20) : {
      | 	pedCycObjCondSuppFlg = true;
      | }
  (junction 22) -> (junction 7)
  (junction 20) -> (junction 22)
  (junction 7) -> (junction 26)
  data: ObjectTypeCameraConfirmed input; objType input Enum: ObjectType; subjCurvTraj input; subjLatAccel input; subjVel input; vehConfigAEBCyc input; vehConfigAEBPed input; AEB_PedResp input; pedCycObjCondSuppFlg output; CNSwtOFF parameter; PsubjVelThres input; PsubjCurvtraijThres input; PsubjLatAccelThres input; subjDrvCondSuppFlg local boolean

== stateflow chart TOS_LIB/StateDelayAbortion/StateDelayAbortion ==
  state NormalState
    en:
    stateOut = state;
    CNTimeCounterMAX = 256;
    Flag=1;
    du:
    stateOut = state;
    Flag=1;
  state CounterState
    en:
    timeSinceLastState = 0;
    Flag=2;
    du:
    timeSinceLastState +=  Ts;
    CounterStateFunc();
    Flag=2;
  state CounterStateFunc [function]
    (default) -> (junction 70)
    (junction 70) -> (junction 62) [order 1] : [timeSinceLastState > CNTimeCounterMAX]
    (junction 70) -> (junction 69) [order 2] : %do nothing
    (junction 62) -> (junction 61) : {
        | 	timeSinceLastState = CNTimeCounterMAX;
        | }
    (junction 61) -> (junction 69)
    (junction 69) -> (junction 68)
    (junction 68) -> (junction 60) [order 1] : [timeSinceLastState < stateProlongationTime]
    (junction 68) -> (junction 66) [order 2] : {
        | 	stateOut = state;
        | }
    (junction 60) -> (junction 67) : {
        | 	stateOut = true;
        | }
    (junction 67) -> (junction 66)
    (junction 66) -> (junction 56)
  (default) -> NormalState
  NormalState -> CounterState : [stateK1 == true &&...
      | state == false]
  CounterState -> NormalState : [timeSinceLastState > stateProlongationTime]
  data: state input; stateK1 input; stateProlongationTime input; timeSinceLastState output double; stateOut output boolean; Ts input; CNTimeCounterMAX local double; Flag output single
